simulink model "six_plus_six_AcmsteeringV09_main"  (R2014a)
settings: Solver=FixedStepDiscrete  StartTime=0.0  StopTime=10.0  FixedStep=0.0005  RelTol=1e-3
InitFcn:
  | Veh_Par_wxt
values from neighbouring files (symbols this model uses):
  acc_spdctl = [0 100]    [Veh_Par_wxt.m]
  ag_thr = ecucoder_cal(ag_thr)    [Veh_Par_wxt.m]
  B = 1.8    [Veh_Par_wxt.m]
  bra_em = 100    [Veh_Par_wxt.m]
  bra_pre_gz2 = 100/3    (= 33.3333333333)    [Veh_Par_wxt.m]
  bra_pre_gz34 = 10/3    (= 3.33333333333)    [Veh_Par_wxt.m]
  bra_pre_yd = 10/2    (= 5)    [Veh_Par_wxt.m]
  brakepre_dem_data = [0 1 2 3 4 5 6 7 8 9 10]    [Veh_Par_wxt.m]
  brakeTrq_dem_data = [0 125 251 376 502 627 753 878 1004 1129 1255]    [Veh_Par_wxt.m]
  bratrq_max = 4*1255    (= 5020)    [Veh_Par_wxt.m]
  eff_tran = 0.9    [Veh_Par_wxt.m]
  ESP_switch = ecucoder_cal(ESP_switch)    [Veh_Par_wxt.m]
  G = Mass*g    (= 15696)    [Veh_Par_wxt.m]
  kd1 = ecucoder_cal(kd1)    [Veh_Par_wxt.m]
  kd2 = 0    [Veh_Par_wxt.m]
  ki1 = ecucoder_cal(ki1)    [Veh_Par_wxt.m]
  ki2 = 1    [Veh_Par_wxt.m]
  kp1 = ecucoder_cal(kp1)    [Veh_Par_wxt.m]
  kp2 = 300    [Veh_Par_wxt.m]
  L = L1+L2    (= 2.9)    [Veh_Par_wxt.m]
  premax = 100    [Veh_Par_wxt.m]
  Radius = 0.4572/2    (= 0.2286)    [Veh_Par_wxt.m]
  RC_switch = ecucoder_cal(RC_switch)    [Veh_Par_wxt.m]
  s_opt_yi = 0.15    [Veh_Par_wxt.m]
  s_opt_zhuan = 0.8    [Veh_Par_wxt.m]
  s_opt_zhuan_add = 0.05    [Veh_Par_wxt.m]
  s_opt_zhuan_table = [0.8 0.8 0.3 0.3]    [Veh_Par_wxt.m]
  spd_map_mot = [0 499.85 999.79 1500 2000 2500 3000 3500 4000 4500 4999.8 5999.8]    [Veh_Par_wxt.m]
  spd_spdctl = [0 500]    [Veh_Par_wxt.m]
  speed_thr_park = 5/3.6/Radius*tras_ratio*30/pi    (= 464.143899364)    [Veh_Par_wxt.m]
  TCS_switch = ecucoder_cal(TCS_switch)    [Veh_Par_wxt.m]
  tras_ratio = 8    [Veh_Par_wxt.m]
  trq_map_mot = [70.5 70.012 71.154 65.797 53.917 45.159 38.073 32.685 27.48 17.133 14.949 10.07]    [Veh_Par_wxt.m]
  trqmax_yd = 70.5    [Veh_Par_wxt.m]
  trqmax_zx = 70.5    [Veh_Par_wxt.m]
  trqmaxneg = -70.5    [Veh_Par_wxt.m]
  v_gain = 0.9    [Veh_Par_wxt.m]
  v_table = [0 5 20 100]    [Veh_Par_wxt.m]
  v_thr_park = 5    [Veh_Par_wxt.m]
  zhidong_bianmazhi = [-140000 750000]    [Veh_Par_wxt.m]
  zhidong_down = -140000    [Veh_Par_wxt.m]
  zhidong_up = 750000    [Veh_Par_wxt.m]
  zhidong_youmen = [0 100]    [Veh_Par_wxt.m]
  zhuanxiang_bianmazhi = [-400000 0 400000]    [Veh_Par_wxt.m]
  zhuanxiang_down = -400000    [Veh_Par_wxt.m]
  zhuanxiang_up = 400000    [Veh_Par_wxt.m]
  zhuanxiang_youmen = [-100 0 100]    [Veh_Par_wxt.m]
undefined symbols (not defined in the file or in its folder): ecucoder_acal, guzhang_lf, guzhang_lm, guzhang_lr, guzhang_rf, guzhang_rm, guzhang_rr, myFIS
libraries: simulink x979, ec5744lib x59, fuzblock x2
(part 16 of 26)

== system six_plus_six_AcmsteeringV09_main/Subsystem/VCU4/VCU1_GearCmd ==
  VCU1_GearCmd : Inport
  Constant{2..8} (7 alike) : Constant  Value=0  OutDataTypeStr=uint8
  VCU1_GearCmdRon : Rounding  Operator=round
  VCU1_GearCmd_1sat : Saturate  UpperLimit=24  LowerLimit=0
  VCU1_GearCmd_Convert : DataTypeConversion  OutDataTypeStr=uint8
  VCU1_GearCmd_Convert1 : DataTypeConversion  OutDataTypeStr=uint32
  VCU1_GearCmd_D : Product  Inputs=*/
  VCU1_GearCmd_F : Constant  OutDataTypeStr=single
  VCU1_GearCmd_L : simulink/Logic and Bit Operations/Bitwise Operator  logicop=AND  UseBitMask=on  BitMask=24  BitMaskRealWorld=Stored Integer
  VCU1_GearCmd_O : Constant  Value=0  OutDataTypeStr=single
  VCU1_GearCmd_S : ArithShift  BitShiftNumber=-3
  VCU1_GearCmd_sat : Saturate  UpperLimit=3  LowerLimit=0
  VCU1_GearCmd_st : Sum  Inputs=+-
  output1 : Outport
  output2 : Outport  Port=2
  output3 : Outport  Port=3
  output4 : Outport  Port=4
  output5 : Outport  Port=5
  output6 : Outport  Port=6
  output7 : Outport  Port=7
  output8 : Outport  Port=8
  wires:
  VCU1_GearCmd/1 -> VCU1_GearCmd_sat/1
  VCU1_GearCmd_sat/1 -> VCU1_GearCmd_st/1
  VCU1_GearCmd_O/1 -> VCU1_GearCmd_st/2
  VCU1_GearCmd_st/1 -> VCU1_GearCmd_D/1
  VCU1_GearCmd_F/1 -> VCU1_GearCmd_D/2
  VCU1_GearCmd_D/1 -> VCU1_GearCmdRon/1
  VCU1_GearCmdRon/1 -> VCU1_GearCmd_S/1
  VCU1_GearCmd_S/1 -> VCU1_GearCmd_1sat/1
  VCU1_GearCmd_1sat/1 -> VCU1_GearCmd_Convert1/1
  VCU1_GearCmd_Convert1/1 -> VCU1_GearCmd_L/1
  VCU1_GearCmd_L/1 -> VCU1_GearCmd_Convert/1
  VCU1_GearCmd_Convert/1 -> output1/1
  Constant2/1 -> output2/1
  Constant3/1 -> output3/1
  Constant4/1 -> output4/1
  Constant5/1 -> output5/1
  Constant6/1 -> output6/1
  Constant7/1 -> output7/1
  Constant8/1 -> output8/1

== system six_plus_six_AcmsteeringV09_main/Subsystem/VCU4/VCU1_LifeCnt ==
  VCU1_LifeCnt : Inport
  Constant{1..7} (7 alike) : Constant  Value=0  OutDataTypeStr=uint8
  VCU1_LifeCntRon : Rounding  Operator=round
  VCU1_LifeCnt_1sat : Saturate  UpperLimit=255  LowerLimit=0
  VCU1_LifeCnt_Convert : DataTypeConversion  OutDataTypeStr=uint8
  VCU1_LifeCnt_Convert1 : DataTypeConversion  OutDataTypeStr=uint32
  VCU1_LifeCnt_D : Product  Inputs=*/
  VCU1_LifeCnt_F : Constant  OutDataTypeStr=single
  VCU1_LifeCnt_L : simulink/Logic and Bit Operations/Bitwise Operator  logicop=AND  UseBitMask=on  BitMask=255  BitMaskRealWorld=Stored Integer
  VCU1_LifeCnt_O : Constant  Value=0  OutDataTypeStr=single
  VCU1_LifeCnt_S : ArithShift
  VCU1_LifeCnt_sat : Saturate  UpperLimit=255  LowerLimit=0
  VCU1_LifeCnt_st : Sum  Inputs=+-
  output1 : Outport
  output2 : Outport  Port=2
  output3 : Outport  Port=3
  output4 : Outport  Port=4
  output5 : Outport  Port=5
  output6 : Outport  Port=6
  output7 : Outport  Port=7
  output8 : Outport  Port=8
  wires:
  VCU1_LifeCnt/1 -> VCU1_LifeCnt_sat/1
  VCU1_LifeCnt_sat/1 -> VCU1_LifeCnt_st/1
  VCU1_LifeCnt_O/1 -> VCU1_LifeCnt_st/2
  VCU1_LifeCnt_st/1 -> VCU1_LifeCnt_D/1
  VCU1_LifeCnt_F/1 -> VCU1_LifeCnt_D/2
  VCU1_LifeCnt_D/1 -> VCU1_LifeCntRon/1
  VCU1_LifeCntRon/1 -> VCU1_LifeCnt_S/1
  VCU1_LifeCnt_S/1 -> VCU1_LifeCnt_1sat/1
  VCU1_LifeCnt_1sat/1 -> VCU1_LifeCnt_Convert1/1
  VCU1_LifeCnt_Convert1/1 -> VCU1_LifeCnt_L/1
  VCU1_LifeCnt_L/1 -> VCU1_LifeCnt_Convert/1
  VCU1_LifeCnt_Convert/1 -> output8/1
  Constant1/1 -> output1/1
  Constant2/1 -> output2/1
  Constant3/1 -> output3/1
  Constant4/1 -> output4/1
  Constant5/1 -> output5/1
  Constant6/1 -> output6/1
  Constant7/1 -> output7/1

== system six_plus_six_AcmsteeringV09_main/Subsystem/VCU4/VCU1_SpeedMax ==
  VCU1_SpeedMax : Inport
  Constant{1,4..8} (6 alike) : Constant  Value=0  OutDataTypeStr=uint8
  VCU1_SpeedMaxBitCov : DataTypeConversion  OutDataTypeStr=uint8
  VCU1_SpeedMaxCOV : DataTypeConversion  OutDataTypeStr=uint8
  VCU1_SpeedMaxRon : Rounding  Operator=round
  VCU1_SpeedMax_1sat : Saturate  UpperLimit=65535  LowerLimit=0
  VCU1_SpeedMax_And : simulink/Logic and Bit Operations/Bitwise Operator  logicop=AND  UseBitMask=off  NumInputPorts=2  BitMask=bin2dec('11011001')  BitMaskRealWorld=Stored Integer
  VCU1_SpeedMax_And_C : Constant  Value=255  OutDataTypeStr=uint32
  VCU1_SpeedMax_Convert : DataTypeConversion  OutDataTypeStr=uint32
  VCU1_SpeedMax_D : Product  Inputs=*/
  VCU1_SpeedMax_D1 : Product  Inputs=*/
  VCU1_SpeedMax_F : Constant  OutDataTypeStr=single
  VCU1_SpeedMax_L : simulink/Logic and Bit Operations/Bitwise Operator  logicop=AND  UseBitMask=on  BitMask=65535  BitMaskRealWorld=Stored Integer
  VCU1_SpeedMax_O : Constant  Value=0  OutDataTypeStr=single
  VCU1_SpeedMax_S : ArithShift
  VCU1_SpeedMax_sat : Saturate  UpperLimit=10000  LowerLimit=0
  VCU1_SpeedMax_st : Sum  Inputs=+-
  VCU1_SpeedMaxoutput2_C : Constant  Value=256
  output1 : Outport
  output2 : Outport  Port=2
  output3 : Outport  Port=3
  output4 : Outport  Port=4
  output5 : Outport  Port=5
  output6 : Outport  Port=6
  output7 : Outport  Port=7
  output8 : Outport  Port=8
  wires:
  VCU1_SpeedMax/1 -> VCU1_SpeedMax_sat/1
  VCU1_SpeedMax_sat/1 -> VCU1_SpeedMax_st/1
  VCU1_SpeedMax_O/1 -> VCU1_SpeedMax_st/2
  VCU1_SpeedMax_st/1 -> VCU1_SpeedMax_D/1
  VCU1_SpeedMax_F/1 -> VCU1_SpeedMax_D/2
  VCU1_SpeedMax_D/1 -> VCU1_SpeedMaxRon/1
  VCU1_SpeedMaxRon/1 -> VCU1_SpeedMax_S/1
  VCU1_SpeedMax_S/1 -> VCU1_SpeedMax_1sat/1
  VCU1_SpeedMax_1sat/1 -> VCU1_SpeedMax_Convert/1
  VCU1_SpeedMax_Convert/1 -> VCU1_SpeedMax_L/1
  VCU1_SpeedMax_L/1 -> VCU1_SpeedMax_D1/1, VCU1_SpeedMax_And/1
  VCU1_SpeedMaxoutput2_C/1 -> VCU1_SpeedMax_D1/2
  VCU1_SpeedMax_D1/1 -> VCU1_SpeedMaxCOV/1
  VCU1_SpeedMaxCOV/1 -> output2/1
  VCU1_SpeedMax_And_C/1 -> VCU1_SpeedMax_And/2
  VCU1_SpeedMax_And/1 -> VCU1_SpeedMaxBitCov/1
  VCU1_SpeedMaxBitCov/1 -> output3/1
  Constant1/1 -> output1/1
  Constant4/1 -> output4/1
  Constant5/1 -> output5/1
  Constant6/1 -> output6/1
  Constant7/1 -> output7/1
  Constant8/1 -> output8/1

== system six_plus_six_AcmsteeringV09_main/Subsystem/VCU4/VCU1_TorqueRef ==
  VCU1_TorqueRef : Inport
  Constant{1..3,6..8} (6 alike) : Constant  Value=0  OutDataTypeStr=uint8
  VCU1_TorqueRefBitCov : DataTypeConversion  OutDataTypeStr=uint8
  VCU1_TorqueRefCOV : DataTypeConversion  OutDataTypeStr=uint8
  VCU1_TorqueRefRon : Rounding  Operator=round
  VCU1_TorqueRef_1sat : Saturate  UpperLimit=65535  LowerLimit=0
  VCU1_TorqueRef_And : simulink/Logic and Bit Operations/Bitwise Operator  logicop=AND  UseBitMask=off  NumInputPorts=2  BitMask=bin2dec('11011001')  BitMaskRealWorld=Stored Integer
  VCU1_TorqueRef_And_C : Constant  Value=255  OutDataTypeStr=uint32
  VCU1_TorqueRef_Convert : DataTypeConversion  OutDataTypeStr=uint32
  VCU1_TorqueRef_D : Product  Inputs=*/
  VCU1_TorqueRef_D1 : Product  Inputs=*/
  VCU1_TorqueRef_F : Constant  Value=0.1  OutDataTypeStr=single
  VCU1_TorqueRef_L : simulink/Logic and Bit Operations/Bitwise Operator  logicop=AND  UseBitMask=on  BitMask=65535  BitMaskRealWorld=Stored Integer
  VCU1_TorqueRef_O : Constant  Value=-1000  OutDataTypeStr=single
  VCU1_TorqueRef_S : ArithShift
  VCU1_TorqueRef_sat : Saturate  UpperLimit=1000  LowerLimit=-1000
  VCU1_TorqueRef_st : Sum  Inputs=+-
  VCU1_TorqueRefoutput4_C : Constant  Value=256
  output1 : Outport
  output2 : Outport  Port=2
  output3 : Outport  Port=3
  output4 : Outport  Port=4
  output5 : Outport  Port=5
  output6 : Outport  Port=6
  output7 : Outport  Port=7
  output8 : Outport  Port=8
  wires:
  VCU1_TorqueRef/1 -> VCU1_TorqueRef_sat/1
  VCU1_TorqueRef_sat/1 -> VCU1_TorqueRef_st/1
  VCU1_TorqueRef_O/1 -> VCU1_TorqueRef_st/2
  VCU1_TorqueRef_st/1 -> VCU1_TorqueRef_D/1
  VCU1_TorqueRef_F/1 -> VCU1_TorqueRef_D/2
  VCU1_TorqueRef_D/1 -> VCU1_TorqueRefRon/1
  VCU1_TorqueRefRon/1 -> VCU1_TorqueRef_S/1
  VCU1_TorqueRef_S/1 -> VCU1_TorqueRef_1sat/1
  VCU1_TorqueRef_1sat/1 -> VCU1_TorqueRef_Convert/1
  VCU1_TorqueRef_Convert/1 -> VCU1_TorqueRef_L/1
  VCU1_TorqueRef_L/1 -> VCU1_TorqueRef_D1/1, VCU1_TorqueRef_And/1
  VCU1_TorqueRefoutput4_C/1 -> VCU1_TorqueRef_D1/2
  VCU1_TorqueRef_D1/1 -> VCU1_TorqueRefCOV/1
  VCU1_TorqueRefCOV/1 -> output4/1
  VCU1_TorqueRef_And_C/1 -> VCU1_TorqueRef_And/2
  VCU1_TorqueRef_And/1 -> VCU1_TorqueRefBitCov/1
  VCU1_TorqueRefBitCov/1 -> output5/1
  Constant1/1 -> output1/1
  Constant2/1 -> output2/1
  Constant3/1 -> output3/1
  Constant6/1 -> output6/1
  Constant7/1 -> output7/1
  Constant8/1 -> output8/1

== system six_plus_six_AcmsteeringV09_main/Subsystem/VCU5/VCU1_CtrlModel ==
  VCU1_CtrlModel : Inport
  Constant{2..8} (7 alike) : Constant  Value=0  OutDataTypeStr=uint8
  VCU1_CtrlModelRon : Rounding  Operator=round
  VCU1_CtrlModel_1sat : Saturate  UpperLimit=4  LowerLimit=0
  VCU1_CtrlModel_Convert : DataTypeConversion  OutDataTypeStr=uint8
  VCU1_CtrlModel_Convert1 : DataTypeConversion  OutDataTypeStr=uint32
  VCU1_CtrlModel_D : Product  Inputs=*/
  VCU1_CtrlModel_F : Constant  OutDataTypeStr=single
  VCU1_CtrlModel_L : simulink/Logic and Bit Operations/Bitwise Operator  logicop=AND  UseBitMask=on  BitMask=4  BitMaskRealWorld=Stored Integer
  VCU1_CtrlModel_O : Constant  Value=0  OutDataTypeStr=single
  VCU1_CtrlModel_S : ArithShift  BitShiftNumber=-2
  VCU1_CtrlModel_sat : Saturate  UpperLimit=1  LowerLimit=0
  VCU1_CtrlModel_st : Sum  Inputs=+-
  output1 : Outport
  output2 : Outport  Port=2
  output3 : Outport  Port=3
  output4 : Outport  Port=4
  output5 : Outport  Port=5
  output6 : Outport  Port=6
  output7 : Outport  Port=7
  output8 : Outport  Port=8
  wires:
  VCU1_CtrlModel/1 -> VCU1_CtrlModel_sat/1
  VCU1_CtrlModel_sat/1 -> VCU1_CtrlModel_st/1
  VCU1_CtrlModel_O/1 -> VCU1_CtrlModel_st/2
  VCU1_CtrlModel_st/1 -> VCU1_CtrlModel_D/1
  VCU1_CtrlModel_F/1 -> VCU1_CtrlModel_D/2
  VCU1_CtrlModel_D/1 -> VCU1_CtrlModelRon/1
  VCU1_CtrlModelRon/1 -> VCU1_CtrlModel_S/1
  VCU1_CtrlModel_S/1 -> VCU1_CtrlModel_1sat/1
  VCU1_CtrlModel_1sat/1 -> VCU1_CtrlModel_Convert1/1
  VCU1_CtrlModel_Convert1/1 -> VCU1_CtrlModel_L/1
  VCU1_CtrlModel_L/1 -> VCU1_CtrlModel_Convert/1
  VCU1_CtrlModel_Convert/1 -> output1/1
  Constant2/1 -> output2/1
  Constant3/1 -> output3/1
  Constant4/1 -> output4/1
  Constant5/1 -> output5/1
  Constant6/1 -> output6/1
  Constant7/1 -> output7/1
  Constant8/1 -> output8/1

== system six_plus_six_AcmsteeringV09_main/Subsystem/VCU5/VCU1_EnableReq ==
  VCU1_EnableReq : Inport
  Constant{2..8} (7 alike) : Constant  Value=0  OutDataTypeStr=uint8
  VCU1_EnableReqRon : Rounding  Operator=round
  VCU1_EnableReq_1sat : Saturate  UpperLimit=3  LowerLimit=0
  VCU1_EnableReq_Convert : DataTypeConversion  OutDataTypeStr=uint8
  VCU1_EnableReq_Convert1 : DataTypeConversion  OutDataTypeStr=uint32
  VCU1_EnableReq_D : Product  Inputs=*/
  VCU1_EnableReq_F : Constant  OutDataTypeStr=single
  VCU1_EnableReq_L : simulink/Logic and Bit Operations/Bitwise Operator  logicop=AND  UseBitMask=on  BitMask=3  BitMaskRealWorld=Stored Integer
  VCU1_EnableReq_O : Constant  Value=0  OutDataTypeStr=single
  VCU1_EnableReq_S : ArithShift
  VCU1_EnableReq_sat : Saturate  UpperLimit=3  LowerLimit=0
  VCU1_EnableReq_st : Sum  Inputs=+-
  output1 : Outport
  output2 : Outport  Port=2
  output3 : Outport  Port=3
  output4 : Outport  Port=4
  output5 : Outport  Port=5
  output6 : Outport  Port=6
  output7 : Outport  Port=7
  output8 : Outport  Port=8
  wires:
  VCU1_EnableReq/1 -> VCU1_EnableReq_sat/1
  VCU1_EnableReq_sat/1 -> VCU1_EnableReq_st/1
  VCU1_EnableReq_O/1 -> VCU1_EnableReq_st/2
  VCU1_EnableReq_st/1 -> VCU1_EnableReq_D/1
  VCU1_EnableReq_F/1 -> VCU1_EnableReq_D/2
  VCU1_EnableReq_D/1 -> VCU1_EnableReqRon/1
  VCU1_EnableReqRon/1 -> VCU1_EnableReq_S/1
  VCU1_EnableReq_S/1 -> VCU1_EnableReq_1sat/1
  VCU1_EnableReq_1sat/1 -> VCU1_EnableReq_Convert1/1
  VCU1_EnableReq_Convert1/1 -> VCU1_EnableReq_L/1
  VCU1_EnableReq_L/1 -> VCU1_EnableReq_Convert/1
  VCU1_EnableReq_Convert/1 -> output1/1
  Constant2/1 -> output2/1
  Constant3/1 -> output3/1
  Constant4/1 -> output4/1
  Constant5/1 -> output5/1
  Constant6/1 -> output6/1
  Constant7/1 -> output7/1
  Constant8/1 -> output8/1

== system six_plus_six_AcmsteeringV09_main/Subsystem/VCU5/VCU1_GearCmd ==
  VCU1_GearCmd : Inport
  Constant{2..8} (7 alike) : Constant  Value=0  OutDataTypeStr=uint8
  VCU1_GearCmdRon : Rounding  Operator=round
  VCU1_GearCmd_1sat : Saturate  UpperLimit=24  LowerLimit=0
  VCU1_GearCmd_Convert : DataTypeConversion  OutDataTypeStr=uint8
  VCU1_GearCmd_Convert1 : DataTypeConversion  OutDataTypeStr=uint32
  VCU1_GearCmd_D : Product  Inputs=*/
  VCU1_GearCmd_F : Constant  OutDataTypeStr=single
  VCU1_GearCmd_L : simulink/Logic and Bit Operations/Bitwise Operator  logicop=AND  UseBitMask=on  BitMask=24  BitMaskRealWorld=Stored Integer
  VCU1_GearCmd_O : Constant  Value=0  OutDataTypeStr=single
  VCU1_GearCmd_S : ArithShift  BitShiftNumber=-3
  VCU1_GearCmd_sat : Saturate  UpperLimit=3  LowerLimit=0
  VCU1_GearCmd_st : Sum  Inputs=+-
  output1 : Outport
  output2 : Outport  Port=2
  output3 : Outport  Port=3
  output4 : Outport  Port=4
  output5 : Outport  Port=5
  output6 : Outport  Port=6
  output7 : Outport  Port=7
  output8 : Outport  Port=8
  wires:
  VCU1_GearCmd/1 -> VCU1_GearCmd_sat/1
  VCU1_GearCmd_sat/1 -> VCU1_GearCmd_st/1
  VCU1_GearCmd_O/1 -> VCU1_GearCmd_st/2
  VCU1_GearCmd_st/1 -> VCU1_GearCmd_D/1
  VCU1_GearCmd_F/1 -> VCU1_GearCmd_D/2
  VCU1_GearCmd_D/1 -> VCU1_GearCmdRon/1
  VCU1_GearCmdRon/1 -> VCU1_GearCmd_S/1
  VCU1_GearCmd_S/1 -> VCU1_GearCmd_1sat/1
  VCU1_GearCmd_1sat/1 -> VCU1_GearCmd_Convert1/1
  VCU1_GearCmd_Convert1/1 -> VCU1_GearCmd_L/1
  VCU1_GearCmd_L/1 -> VCU1_GearCmd_Convert/1
  VCU1_GearCmd_Convert/1 -> output1/1
  Constant2/1 -> output2/1
  Constant3/1 -> output3/1
  Constant4/1 -> output4/1
  Constant5/1 -> output5/1
  Constant6/1 -> output6/1
  Constant7/1 -> output7/1
  Constant8/1 -> output8/1

== system six_plus_six_AcmsteeringV09_main/Subsystem/VCU5/VCU1_LifeCnt ==
  VCU1_LifeCnt : Inport
  Constant{1..7} (7 alike) : Constant  Value=0  OutDataTypeStr=uint8
  VCU1_LifeCntRon : Rounding  Operator=round
  VCU1_LifeCnt_1sat : Saturate  UpperLimit=255  LowerLimit=0
  VCU1_LifeCnt_Convert : DataTypeConversion  OutDataTypeStr=uint8
  VCU1_LifeCnt_Convert1 : DataTypeConversion  OutDataTypeStr=uint32
  VCU1_LifeCnt_D : Product  Inputs=*/
  VCU1_LifeCnt_F : Constant  OutDataTypeStr=single
  VCU1_LifeCnt_L : simulink/Logic and Bit Operations/Bitwise Operator  logicop=AND  UseBitMask=on  BitMask=255  BitMaskRealWorld=Stored Integer
  VCU1_LifeCnt_O : Constant  Value=0  OutDataTypeStr=single
  VCU1_LifeCnt_S : ArithShift
  VCU1_LifeCnt_sat : Saturate  UpperLimit=255  LowerLimit=0
  VCU1_LifeCnt_st : Sum  Inputs=+-
  output1 : Outport
  output2 : Outport  Port=2
  output3 : Outport  Port=3
  output4 : Outport  Port=4
  output5 : Outport  Port=5
  output6 : Outport  Port=6
  output7 : Outport  Port=7
  output8 : Outport  Port=8
  wires:
  VCU1_LifeCnt/1 -> VCU1_LifeCnt_sat/1
  VCU1_LifeCnt_sat/1 -> VCU1_LifeCnt_st/1
  VCU1_LifeCnt_O/1 -> VCU1_LifeCnt_st/2
  VCU1_LifeCnt_st/1 -> VCU1_LifeCnt_D/1
  VCU1_LifeCnt_F/1 -> VCU1_LifeCnt_D/2
  VCU1_LifeCnt_D/1 -> VCU1_LifeCntRon/1
  VCU1_LifeCntRon/1 -> VCU1_LifeCnt_S/1
  VCU1_LifeCnt_S/1 -> VCU1_LifeCnt_1sat/1
  VCU1_LifeCnt_1sat/1 -> VCU1_LifeCnt_Convert1/1
  VCU1_LifeCnt_Convert1/1 -> VCU1_LifeCnt_L/1
  VCU1_LifeCnt_L/1 -> VCU1_LifeCnt_Convert/1
  VCU1_LifeCnt_Convert/1 -> output8/1
  Constant1/1 -> output1/1
  Constant2/1 -> output2/1
  Constant3/1 -> output3/1
  Constant4/1 -> output4/1
  Constant5/1 -> output5/1
  Constant6/1 -> output6/1
  Constant7/1 -> output7/1

== system six_plus_six_AcmsteeringV09_main/Subsystem/VCU5/VCU1_SpeedMax ==
  VCU1_SpeedMax : Inport
  Constant{1,4..8} (6 alike) : Constant  Value=0  OutDataTypeStr=uint8
  VCU1_SpeedMaxBitCov : DataTypeConversion  OutDataTypeStr=uint8
  VCU1_SpeedMaxCOV : DataTypeConversion  OutDataTypeStr=uint8
  VCU1_SpeedMaxRon : Rounding  Operator=round
  VCU1_SpeedMax_1sat : Saturate  UpperLimit=65535  LowerLimit=0
  VCU1_SpeedMax_And : simulink/Logic and Bit Operations/Bitwise Operator  logicop=AND  UseBitMask=off  NumInputPorts=2  BitMask=bin2dec('11011001')  BitMaskRealWorld=Stored Integer
  VCU1_SpeedMax_And_C : Constant  Value=255  OutDataTypeStr=uint32
  VCU1_SpeedMax_Convert : DataTypeConversion  OutDataTypeStr=uint32
  VCU1_SpeedMax_D : Product  Inputs=*/
  VCU1_SpeedMax_D1 : Product  Inputs=*/
  VCU1_SpeedMax_F : Constant  OutDataTypeStr=single
  VCU1_SpeedMax_L : simulink/Logic and Bit Operations/Bitwise Operator  logicop=AND  UseBitMask=on  BitMask=65535  BitMaskRealWorld=Stored Integer
  VCU1_SpeedMax_O : Constant  Value=0  OutDataTypeStr=single
  VCU1_SpeedMax_S : ArithShift
  VCU1_SpeedMax_sat : Saturate  UpperLimit=10000  LowerLimit=0
  VCU1_SpeedMax_st : Sum  Inputs=+-
  VCU1_SpeedMaxoutput2_C : Constant  Value=256
  output1 : Outport
  output2 : Outport  Port=2
  output3 : Outport  Port=3
  output4 : Outport  Port=4
  output5 : Outport  Port=5
  output6 : Outport  Port=6
  output7 : Outport  Port=7
  output8 : Outport  Port=8
  wires:
  VCU1_SpeedMax/1 -> VCU1_SpeedMax_sat/1
  VCU1_SpeedMax_sat/1 -> VCU1_SpeedMax_st/1
  VCU1_SpeedMax_O/1 -> VCU1_SpeedMax_st/2
  VCU1_SpeedMax_st/1 -> VCU1_SpeedMax_D/1
  VCU1_SpeedMax_F/1 -> VCU1_SpeedMax_D/2
  VCU1_SpeedMax_D/1 -> VCU1_SpeedMaxRon/1
  VCU1_SpeedMaxRon/1 -> VCU1_SpeedMax_S/1
  VCU1_SpeedMax_S/1 -> VCU1_SpeedMax_1sat/1
  VCU1_SpeedMax_1sat/1 -> VCU1_SpeedMax_Convert/1
  VCU1_SpeedMax_Convert/1 -> VCU1_SpeedMax_L/1
  VCU1_SpeedMax_L/1 -> VCU1_SpeedMax_D1/1, VCU1_SpeedMax_And/1
  VCU1_SpeedMaxoutput2_C/1 -> VCU1_SpeedMax_D1/2
  VCU1_SpeedMax_D1/1 -> VCU1_SpeedMaxCOV/1
  VCU1_SpeedMaxCOV/1 -> output2/1
  VCU1_SpeedMax_And_C/1 -> VCU1_SpeedMax_And/2
  VCU1_SpeedMax_And/1 -> VCU1_SpeedMaxBitCov/1
  VCU1_SpeedMaxBitCov/1 -> output3/1
  Constant1/1 -> output1/1
  Constant4/1 -> output4/1
  Constant5/1 -> output5/1
  Constant6/1 -> output6/1
  Constant7/1 -> output7/1
  Constant8/1 -> output8/1

== system six_plus_six_AcmsteeringV09_main/Subsystem/VCU5/VCU1_TorqueRef ==
  VCU1_TorqueRef : Inport
  Constant{1..3,6..8} (6 alike) : Constant  Value=0  OutDataTypeStr=uint8
  VCU1_TorqueRefBitCov : DataTypeConversion  OutDataTypeStr=uint8
  VCU1_TorqueRefCOV : DataTypeConversion  OutDataTypeStr=uint8
  VCU1_TorqueRefRon : Rounding  Operator=round
  VCU1_TorqueRef_1sat : Saturate  UpperLimit=65535  LowerLimit=0
  VCU1_TorqueRef_And : simulink/Logic and Bit Operations/Bitwise Operator  logicop=AND  UseBitMask=off  NumInputPorts=2  BitMask=bin2dec('11011001')  BitMaskRealWorld=Stored Integer
  VCU1_TorqueRef_And_C : Constant  Value=255  OutDataTypeStr=uint32
  VCU1_TorqueRef_Convert : DataTypeConversion  OutDataTypeStr=uint32
  VCU1_TorqueRef_D : Product  Inputs=*/
  VCU1_TorqueRef_D1 : Product  Inputs=*/
  VCU1_TorqueRef_F : Constant  Value=0.1  OutDataTypeStr=single
  VCU1_TorqueRef_L : simulink/Logic and Bit Operations/Bitwise Operator  logicop=AND  UseBitMask=on  BitMask=65535  BitMaskRealWorld=Stored Integer
  VCU1_TorqueRef_O : Constant  Value=-1000  OutDataTypeStr=single
  VCU1_TorqueRef_S : ArithShift
  VCU1_TorqueRef_sat : Saturate  UpperLimit=1000  LowerLimit=-1000
  VCU1_TorqueRef_st : Sum  Inputs=+-
  VCU1_TorqueRefoutput4_C : Constant  Value=256
  output1 : Outport
  output2 : Outport  Port=2
  output3 : Outport  Port=3
  output4 : Outport  Port=4
  output5 : Outport  Port=5
  output6 : Outport  Port=6
  output7 : Outport  Port=7
  output8 : Outport  Port=8
  wires:
  VCU1_TorqueRef/1 -> VCU1_TorqueRef_sat/1
  VCU1_TorqueRef_sat/1 -> VCU1_TorqueRef_st/1
  VCU1_TorqueRef_O/1 -> VCU1_TorqueRef_st/2
  VCU1_TorqueRef_st/1 -> VCU1_TorqueRef_D/1
  VCU1_TorqueRef_F/1 -> VCU1_TorqueRef_D/2
  VCU1_TorqueRef_D/1 -> VCU1_TorqueRefRon/1
  VCU1_TorqueRefRon/1 -> VCU1_TorqueRef_S/1
  VCU1_TorqueRef_S/1 -> VCU1_TorqueRef_1sat/1
  VCU1_TorqueRef_1sat/1 -> VCU1_TorqueRef_Convert/1
  VCU1_TorqueRef_Convert/1 -> VCU1_TorqueRef_L/1
  VCU1_TorqueRef_L/1 -> VCU1_TorqueRef_D1/1, VCU1_TorqueRef_And/1
  VCU1_TorqueRefoutput4_C/1 -> VCU1_TorqueRef_D1/2
  VCU1_TorqueRef_D1/1 -> VCU1_TorqueRefCOV/1
  VCU1_TorqueRefCOV/1 -> output4/1
  VCU1_TorqueRef_And_C/1 -> VCU1_TorqueRef_And/2
  VCU1_TorqueRef_And/1 -> VCU1_TorqueRefBitCov/1
  VCU1_TorqueRefBitCov/1 -> output5/1
  Constant1/1 -> output1/1
  Constant2/1 -> output2/1
  Constant3/1 -> output3/1
  Constant6/1 -> output6/1
  Constant7/1 -> output7/1
  Constant8/1 -> output8/1

== system six_plus_six_AcmsteeringV09_main/Subsystem/VCU6/VCU1_CtrlModel ==
  VCU1_CtrlModel : Inport
  Constant{2..8} (7 alike) : Constant  Value=0  OutDataTypeStr=uint8
  VCU1_CtrlModelRon : Rounding  Operator=round
  VCU1_CtrlModel_1sat : Saturate  UpperLimit=4  LowerLimit=0
  VCU1_CtrlModel_Convert : DataTypeConversion  OutDataTypeStr=uint8
  VCU1_CtrlModel_Convert1 : DataTypeConversion  OutDataTypeStr=uint32
  VCU1_CtrlModel_D : Product  Inputs=*/
  VCU1_CtrlModel_F : Constant  OutDataTypeStr=single
  VCU1_CtrlModel_L : simulink/Logic and Bit Operations/Bitwise Operator  logicop=AND  UseBitMask=on  BitMask=4  BitMaskRealWorld=Stored Integer
  VCU1_CtrlModel_O : Constant  Value=0  OutDataTypeStr=single
  VCU1_CtrlModel_S : ArithShift  BitShiftNumber=-2
  VCU1_CtrlModel_sat : Saturate  UpperLimit=1  LowerLimit=0
  VCU1_CtrlModel_st : Sum  Inputs=+-
  output1 : Outport
  output2 : Outport  Port=2
  output3 : Outport  Port=3
  output4 : Outport  Port=4
  output5 : Outport  Port=5
  output6 : Outport  Port=6
  output7 : Outport  Port=7
  output8 : Outport  Port=8
  wires:
  VCU1_CtrlModel/1 -> VCU1_CtrlModel_sat/1
  VCU1_CtrlModel_sat/1 -> VCU1_CtrlModel_st/1
  VCU1_CtrlModel_O/1 -> VCU1_CtrlModel_st/2
  VCU1_CtrlModel_st/1 -> VCU1_CtrlModel_D/1
  VCU1_CtrlModel_F/1 -> VCU1_CtrlModel_D/2
  VCU1_CtrlModel_D/1 -> VCU1_CtrlModelRon/1
  VCU1_CtrlModelRon/1 -> VCU1_CtrlModel_S/1
  VCU1_CtrlModel_S/1 -> VCU1_CtrlModel_1sat/1
  VCU1_CtrlModel_1sat/1 -> VCU1_CtrlModel_Convert1/1
  VCU1_CtrlModel_Convert1/1 -> VCU1_CtrlModel_L/1
  VCU1_CtrlModel_L/1 -> VCU1_CtrlModel_Convert/1
  VCU1_CtrlModel_Convert/1 -> output1/1
  Constant2/1 -> output2/1
  Constant3/1 -> output3/1
  Constant4/1 -> output4/1
  Constant5/1 -> output5/1
  Constant6/1 -> output6/1
  Constant7/1 -> output7/1
  Constant8/1 -> output8/1

== system six_plus_six_AcmsteeringV09_main/Subsystem/VCU6/VCU1_EnableReq ==
  VCU1_EnableReq : Inport
  Constant{2..8} (7 alike) : Constant  Value=0  OutDataTypeStr=uint8
  VCU1_EnableReqRon : Rounding  Operator=round
  VCU1_EnableReq_1sat : Saturate  UpperLimit=3  LowerLimit=0
  VCU1_EnableReq_Convert : DataTypeConversion  OutDataTypeStr=uint8
  VCU1_EnableReq_Convert1 : DataTypeConversion  OutDataTypeStr=uint32
  VCU1_EnableReq_D : Product  Inputs=*/
  VCU1_EnableReq_F : Constant  OutDataTypeStr=single
  VCU1_EnableReq_L : simulink/Logic and Bit Operations/Bitwise Operator  logicop=AND  UseBitMask=on  BitMask=3  BitMaskRealWorld=Stored Integer
  VCU1_EnableReq_O : Constant  Value=0  OutDataTypeStr=single
  VCU1_EnableReq_S : ArithShift
  VCU1_EnableReq_sat : Saturate  UpperLimit=3  LowerLimit=0
  VCU1_EnableReq_st : Sum  Inputs=+-
  output1 : Outport
  output2 : Outport  Port=2
  output3 : Outport  Port=3
  output4 : Outport  Port=4
  output5 : Outport  Port=5
  output6 : Outport  Port=6
  output7 : Outport  Port=7
  output8 : Outport  Port=8
  wires:
  VCU1_EnableReq/1 -> VCU1_EnableReq_sat/1
  VCU1_EnableReq_sat/1 -> VCU1_EnableReq_st/1
  VCU1_EnableReq_O/1 -> VCU1_EnableReq_st/2
  VCU1_EnableReq_st/1 -> VCU1_EnableReq_D/1
  VCU1_EnableReq_F/1 -> VCU1_EnableReq_D/2
  VCU1_EnableReq_D/1 -> VCU1_EnableReqRon/1
  VCU1_EnableReqRon/1 -> VCU1_EnableReq_S/1
  VCU1_EnableReq_S/1 -> VCU1_EnableReq_1sat/1
  VCU1_EnableReq_1sat/1 -> VCU1_EnableReq_Convert1/1
  VCU1_EnableReq_Convert1/1 -> VCU1_EnableReq_L/1
  VCU1_EnableReq_L/1 -> VCU1_EnableReq_Convert/1
  VCU1_EnableReq_Convert/1 -> output1/1
  Constant2/1 -> output2/1
  Constant3/1 -> output3/1
  Constant4/1 -> output4/1
  Constant5/1 -> output5/1
  Constant6/1 -> output6/1
  Constant7/1 -> output7/1
  Constant8/1 -> output8/1

== system six_plus_six_AcmsteeringV09_main/Subsystem/VCU6/VCU1_GearCmd ==
  VCU1_GearCmd : Inport
  Constant{2..8} (7 alike) : Constant  Value=0  OutDataTypeStr=uint8
  VCU1_GearCmdRon : Rounding  Operator=round
  VCU1_GearCmd_1sat : Saturate  UpperLimit=24  LowerLimit=0
  VCU1_GearCmd_Convert : DataTypeConversion  OutDataTypeStr=uint8
  VCU1_GearCmd_Convert1 : DataTypeConversion  OutDataTypeStr=uint32
  VCU1_GearCmd_D : Product  Inputs=*/
  VCU1_GearCmd_F : Constant  OutDataTypeStr=single
  VCU1_GearCmd_L : simulink/Logic and Bit Operations/Bitwise Operator  logicop=AND  UseBitMask=on  BitMask=24  BitMaskRealWorld=Stored Integer
  VCU1_GearCmd_O : Constant  Value=0  OutDataTypeStr=single
  VCU1_GearCmd_S : ArithShift  BitShiftNumber=-3
  VCU1_GearCmd_sat : Saturate  UpperLimit=3  LowerLimit=0
  VCU1_GearCmd_st : Sum  Inputs=+-
  output1 : Outport
  output2 : Outport  Port=2
  output3 : Outport  Port=3
  output4 : Outport  Port=4
  output5 : Outport  Port=5
  output6 : Outport  Port=6
  output7 : Outport  Port=7
  output8 : Outport  Port=8
  wires:
  VCU1_GearCmd/1 -> VCU1_GearCmd_sat/1
  VCU1_GearCmd_sat/1 -> VCU1_GearCmd_st/1
  VCU1_GearCmd_O/1 -> VCU1_GearCmd_st/2
  VCU1_GearCmd_st/1 -> VCU1_GearCmd_D/1
  VCU1_GearCmd_F/1 -> VCU1_GearCmd_D/2
  VCU1_GearCmd_D/1 -> VCU1_GearCmdRon/1
  VCU1_GearCmdRon/1 -> VCU1_GearCmd_S/1
  VCU1_GearCmd_S/1 -> VCU1_GearCmd_1sat/1
  VCU1_GearCmd_1sat/1 -> VCU1_GearCmd_Convert1/1
  VCU1_GearCmd_Convert1/1 -> VCU1_GearCmd_L/1
  VCU1_GearCmd_L/1 -> VCU1_GearCmd_Convert/1
  VCU1_GearCmd_Convert/1 -> output1/1
  Constant2/1 -> output2/1
  Constant3/1 -> output3/1
  Constant4/1 -> output4/1
  Constant5/1 -> output5/1
  Constant6/1 -> output6/1
  Constant7/1 -> output7/1
  Constant8/1 -> output8/1

== system six_plus_six_AcmsteeringV09_main/Subsystem/VCU6/VCU1_LifeCnt ==
  VCU1_LifeCnt : Inport
  Constant{1..7} (7 alike) : Constant  Value=0  OutDataTypeStr=uint8
  VCU1_LifeCntRon : Rounding  Operator=round
  VCU1_LifeCnt_1sat : Saturate  UpperLimit=255  LowerLimit=0
  VCU1_LifeCnt_Convert : DataTypeConversion  OutDataTypeStr=uint8
  VCU1_LifeCnt_Convert1 : DataTypeConversion  OutDataTypeStr=uint32
  VCU1_LifeCnt_D : Product  Inputs=*/
  VCU1_LifeCnt_F : Constant  OutDataTypeStr=single
  VCU1_LifeCnt_L : simulink/Logic and Bit Operations/Bitwise Operator  logicop=AND  UseBitMask=on  BitMask=255  BitMaskRealWorld=Stored Integer
  VCU1_LifeCnt_O : Constant  Value=0  OutDataTypeStr=single
  VCU1_LifeCnt_S : ArithShift
  VCU1_LifeCnt_sat : Saturate  UpperLimit=255  LowerLimit=0
  VCU1_LifeCnt_st : Sum  Inputs=+-
  output1 : Outport
  output2 : Outport  Port=2
  output3 : Outport  Port=3
  output4 : Outport  Port=4
  output5 : Outport  Port=5
  output6 : Outport  Port=6
  output7 : Outport  Port=7
  output8 : Outport  Port=8
  wires:
  VCU1_LifeCnt/1 -> VCU1_LifeCnt_sat/1
  VCU1_LifeCnt_sat/1 -> VCU1_LifeCnt_st/1
  VCU1_LifeCnt_O/1 -> VCU1_LifeCnt_st/2
  VCU1_LifeCnt_st/1 -> VCU1_LifeCnt_D/1
  VCU1_LifeCnt_F/1 -> VCU1_LifeCnt_D/2
  VCU1_LifeCnt_D/1 -> VCU1_LifeCntRon/1
  VCU1_LifeCntRon/1 -> VCU1_LifeCnt_S/1
  VCU1_LifeCnt_S/1 -> VCU1_LifeCnt_1sat/1
  VCU1_LifeCnt_1sat/1 -> VCU1_LifeCnt_Convert1/1
  VCU1_LifeCnt_Convert1/1 -> VCU1_LifeCnt_L/1
  VCU1_LifeCnt_L/1 -> VCU1_LifeCnt_Convert/1
  VCU1_LifeCnt_Convert/1 -> output8/1
  Constant1/1 -> output1/1
  Constant2/1 -> output2/1
  Constant3/1 -> output3/1
  Constant4/1 -> output4/1
  Constant5/1 -> output5/1
  Constant6/1 -> output6/1
  Constant7/1 -> output7/1

== system six_plus_six_AcmsteeringV09_main/Subsystem/VCU6/VCU1_SpeedMax ==
  VCU1_SpeedMax : Inport
  Constant{1,4..8} (6 alike) : Constant  Value=0  OutDataTypeStr=uint8
  VCU1_SpeedMaxBitCov : DataTypeConversion  OutDataTypeStr=uint8
  VCU1_SpeedMaxCOV : DataTypeConversion  OutDataTypeStr=uint8
  VCU1_SpeedMaxRon : Rounding  Operator=round
  VCU1_SpeedMax_1sat : Saturate  UpperLimit=65535  LowerLimit=0
  VCU1_SpeedMax_And : simulink/Logic and Bit Operations/Bitwise Operator  logicop=AND  UseBitMask=off  NumInputPorts=2  BitMask=bin2dec('11011001')  BitMaskRealWorld=Stored Integer
  VCU1_SpeedMax_And_C : Constant  Value=255  OutDataTypeStr=uint32
  VCU1_SpeedMax_Convert : DataTypeConversion  OutDataTypeStr=uint32
  VCU1_SpeedMax_D : Product  Inputs=*/
  VCU1_SpeedMax_D1 : Product  Inputs=*/
  VCU1_SpeedMax_F : Constant  OutDataTypeStr=single
  VCU1_SpeedMax_L : simulink/Logic and Bit Operations/Bitwise Operator  logicop=AND  UseBitMask=on  BitMask=65535  BitMaskRealWorld=Stored Integer
  VCU1_SpeedMax_O : Constant  Value=0  OutDataTypeStr=single
  VCU1_SpeedMax_S : ArithShift
  VCU1_SpeedMax_sat : Saturate  UpperLimit=10000  LowerLimit=0
  VCU1_SpeedMax_st : Sum  Inputs=+-
  VCU1_SpeedMaxoutput2_C : Constant  Value=256
  output1 : Outport
  output2 : Outport  Port=2
  output3 : Outport  Port=3
  output4 : Outport  Port=4
  output5 : Outport  Port=5
  output6 : Outport  Port=6
  output7 : Outport  Port=7
  output8 : Outport  Port=8
  wires:
  VCU1_SpeedMax/1 -> VCU1_SpeedMax_sat/1
  VCU1_SpeedMax_sat/1 -> VCU1_SpeedMax_st/1
  VCU1_SpeedMax_O/1 -> VCU1_SpeedMax_st/2
  VCU1_SpeedMax_st/1 -> VCU1_SpeedMax_D/1
  VCU1_SpeedMax_F/1 -> VCU1_SpeedMax_D/2
  VCU1_SpeedMax_D/1 -> VCU1_SpeedMaxRon/1
  VCU1_SpeedMaxRon/1 -> VCU1_SpeedMax_S/1
  VCU1_SpeedMax_S/1 -> VCU1_SpeedMax_1sat/1
  VCU1_SpeedMax_1sat/1 -> VCU1_SpeedMax_Convert/1
  VCU1_SpeedMax_Convert/1 -> VCU1_SpeedMax_L/1
  VCU1_SpeedMax_L/1 -> VCU1_SpeedMax_D1/1, VCU1_SpeedMax_And/1
  VCU1_SpeedMaxoutput2_C/1 -> VCU1_SpeedMax_D1/2
  VCU1_SpeedMax_D1/1 -> VCU1_SpeedMaxCOV/1
  VCU1_SpeedMaxCOV/1 -> output2/1
  VCU1_SpeedMax_And_C/1 -> VCU1_SpeedMax_And/2
  VCU1_SpeedMax_And/1 -> VCU1_SpeedMaxBitCov/1
  VCU1_SpeedMaxBitCov/1 -> output3/1
  Constant1/1 -> output1/1
  Constant4/1 -> output4/1
  Constant5/1 -> output5/1
  Constant6/1 -> output6/1
  Constant7/1 -> output7/1
  Constant8/1 -> output8/1

== system six_plus_six_AcmsteeringV09_main/Subsystem/VCU6/VCU1_TorqueRef ==
  VCU1_TorqueRef : Inport
  Constant{1..3,6..8} (6 alike) : Constant  Value=0  OutDataTypeStr=uint8
  VCU1_TorqueRefBitCov : DataTypeConversion  OutDataTypeStr=uint8
  VCU1_TorqueRefCOV : DataTypeConversion  OutDataTypeStr=uint8
  VCU1_TorqueRefRon : Rounding  Operator=round
  VCU1_TorqueRef_1sat : Saturate  UpperLimit=65535  LowerLimit=0
  VCU1_TorqueRef_And : simulink/Logic and Bit Operations/Bitwise Operator  logicop=AND  UseBitMask=off  NumInputPorts=2  BitMask=bin2dec('11011001')  BitMaskRealWorld=Stored Integer
  VCU1_TorqueRef_And_C : Constant  Value=255  OutDataTypeStr=uint32
  VCU1_TorqueRef_Convert : DataTypeConversion  OutDataTypeStr=uint32
  VCU1_TorqueRef_D : Product  Inputs=*/
  VCU1_TorqueRef_D1 : Product  Inputs=*/
  VCU1_TorqueRef_F : Constant  Value=0.1  OutDataTypeStr=single
  VCU1_TorqueRef_L : simulink/Logic and Bit Operations/Bitwise Operator  logicop=AND  UseBitMask=on  BitMask=65535  BitMaskRealWorld=Stored Integer
  VCU1_TorqueRef_O : Constant  Value=-1000  OutDataTypeStr=single
  VCU1_TorqueRef_S : ArithShift
  VCU1_TorqueRef_sat : Saturate  UpperLimit=1000  LowerLimit=-1000
  VCU1_TorqueRef_st : Sum  Inputs=+-
  VCU1_TorqueRefoutput4_C : Constant  Value=256
  output1 : Outport
  output2 : Outport  Port=2
  output3 : Outport  Port=3
  output4 : Outport  Port=4
  output5 : Outport  Port=5
  output6 : Outport  Port=6
  output7 : Outport  Port=7
  output8 : Outport  Port=8
  wires:
  VCU1_TorqueRef/1 -> VCU1_TorqueRef_sat/1
  VCU1_TorqueRef_sat/1 -> VCU1_TorqueRef_st/1
  VCU1_TorqueRef_O/1 -> VCU1_TorqueRef_st/2
  VCU1_TorqueRef_st/1 -> VCU1_TorqueRef_D/1
  VCU1_TorqueRef_F/1 -> VCU1_TorqueRef_D/2
  VCU1_TorqueRef_D/1 -> VCU1_TorqueRefRon/1
  VCU1_TorqueRefRon/1 -> VCU1_TorqueRef_S/1
  VCU1_TorqueRef_S/1 -> VCU1_TorqueRef_1sat/1
  VCU1_TorqueRef_1sat/1 -> VCU1_TorqueRef_Convert/1
  VCU1_TorqueRef_Convert/1 -> VCU1_TorqueRef_L/1
  VCU1_TorqueRef_L/1 -> VCU1_TorqueRef_D1/1, VCU1_TorqueRef_And/1
  VCU1_TorqueRefoutput4_C/1 -> VCU1_TorqueRef_D1/2
  VCU1_TorqueRef_D1/1 -> VCU1_TorqueRefCOV/1
  VCU1_TorqueRefCOV/1 -> output4/1
  VCU1_TorqueRef_And_C/1 -> VCU1_TorqueRef_And/2
  VCU1_TorqueRef_And/1 -> VCU1_TorqueRefBitCov/1
  VCU1_TorqueRefBitCov/1 -> output5/1
  Constant1/1 -> output1/1
  Constant2/1 -> output2/1
  Constant3/1 -> output3/1
  Constant6/1 -> output6/1
  Constant7/1 -> output7/1
  Constant8/1 -> output8/1

== system six_plus_six_AcmsteeringV09_main/Data_input/BMS1/BMS1/BMS1_SOC_Sub ==
  In1 : Inport
  Out1 : Outport
  wires:
  In1/1 -> Out1/1

== system six_plus_six_AcmsteeringV09_main/Data_input/BMS1/BMS1/BMS1_Sys_Status1_Sub ==
  In1 : Inport
  Out1 : Outport
  wires:
  In1/1 -> Out1/1

== system six_plus_six_AcmsteeringV09_main/Data_input/BMS1/BMS1/BMS1_Sys_Status2_Sub ==
  In1 : Inport
  Out1 : Outport
  wires:
  In1/1 -> Out1/1

== system six_plus_six_AcmsteeringV09_main/Data_input/BMS1/BMS1/BMS1_TotalCurrent_Sub ==
  In1 : Inport
  Out1 : Outport
  wires:
  In1/1 -> Out1/1

== system six_plus_six_AcmsteeringV09_main/Data_input/BMS1/BMS1/BMS1_TotalVol_Sub ==
  In1 : Inport
  Out1 : Outport
  wires:
  In1/1 -> Out1/1

== system six_plus_six_AcmsteeringV09_main/Data_input/BMS1-2/BMS1/BMS1_SOC_Sub ==
  In1 : Inport
  Out1 : Outport
  wires:
  In1/1 -> Out1/1

== system six_plus_six_AcmsteeringV09_main/Data_input/BMS1-2/BMS1/BMS1_Sys_Status1_Sub ==
  In1 : Inport
  Out1 : Outport
  wires:
  In1/1 -> Out1/1

== system six_plus_six_AcmsteeringV09_main/Data_input/BMS1-2/BMS1/BMS1_Sys_Status2_Sub ==
  In1 : Inport
  Out1 : Outport
  wires:
  In1/1 -> Out1/1

== system six_plus_six_AcmsteeringV09_main/Data_input/BMS1-2/BMS1/BMS1_TotalCurrent_Sub ==
  In1 : Inport
  Out1 : Outport
  wires:
  In1/1 -> Out1/1

== system six_plus_six_AcmsteeringV09_main/Data_input/BMS1-2/BMS1/BMS1_TotalVol_Sub ==
  In1 : Inport
  Out1 : Outport
  wires:
  In1/1 -> Out1/1

== system six_plus_six_AcmsteeringV09_main/Data_input/BMS1_1/BMS1/BMS1_SOC_Sub ==
  In1 : Inport
  Out1 : Outport
  wires:
  In1/1 -> Out1/1

== system six_plus_six_AcmsteeringV09_main/Data_input/BMS1_1/BMS1/BMS1_Sys_Status1_Sub ==
  In1 : Inport
  Out1 : Outport
  wires:
  In1/1 -> Out1/1

== system six_plus_six_AcmsteeringV09_main/Data_input/BMS1_1/BMS1/BMS1_Sys_Status2_Sub ==
  In1 : Inport
  Out1 : Outport
  wires:
  In1/1 -> Out1/1

== system six_plus_six_AcmsteeringV09_main/Data_input/BMS1_1/BMS1/BMS1_TotalCurrent_Sub ==
  In1 : Inport
  Out1 : Outport
  wires:
  In1/1 -> Out1/1

== system six_plus_six_AcmsteeringV09_main/Data_input/BMS1_1/BMS1/BMS1_TotalVol_Sub ==
  In1 : Inport
  Out1 : Outport
  wires:
  In1/1 -> Out1/1

== system six_plus_six_AcmsteeringV09_main/Data_input/BMS2/BMS2/BMS2_HighSingleVol_Sub ==
  In1 : Inport
  Out1 : Outport
  wires:
  In1/1 -> Out1/1

== system six_plus_six_AcmsteeringV09_main/Data_input/BMS2/BMS2/BMS2_LowSingleVol_Sub ==
  In1 : Inport
  Out1 : Outport
  wires:
  In1/1 -> Out1/1

== system six_plus_six_AcmsteeringV09_main/Data_input/BMS2_1/BMS2/BMS2_HighSingleVol_Sub ==
  In1 : Inport
  Out1 : Outport
  wires:
  In1/1 -> Out1/1

== system six_plus_six_AcmsteeringV09_main/Data_input/BMS2_1/BMS2/BMS2_LowSingleVol_Sub ==
  In1 : Inport
  Out1 : Outport
  wires:
  In1/1 -> Out1/1

== system six_plus_six_AcmsteeringV09_main/Data_input/BMS2_2/BMS2/BMS2_HighSingleVol_Sub ==
  In1 : Inport
  Out1 : Outport
  wires:
  In1/1 -> Out1/1

== system six_plus_six_AcmsteeringV09_main/Data_input/BMS2_2/BMS2/BMS2_LowSingleVol_Sub ==
  In1 : Inport
  Out1 : Outport
  wires:
  In1/1 -> Out1/1

== system six_plus_six_AcmsteeringV09_main/Data_input/BMS3/BMS3/BMS3_HighTemperature_Sub ==
  In1 : Inport
  Out1 : Outport
  wires:
  In1/1 -> Out1/1

== system six_plus_six_AcmsteeringV09_main/Data_input/BMS3/BMS3/BMS3_LowTemperature_Sub ==
  In1 : Inport
  Out1 : Outport
  wires:
  In1/1 -> Out1/1

== system six_plus_six_AcmsteeringV09_main/Data_input/BMS3_1/BMS3/BMS3_HighTemperature_Sub ==
  In1 : Inport
  Out1 : Outport
  wires:
  In1/1 -> Out1/1

== system six_plus_six_AcmsteeringV09_main/Data_input/BMS3_1/BMS3/BMS3_LowTemperature_Sub ==
  In1 : Inport
  Out1 : Outport
  wires:
  In1/1 -> Out1/1

== system six_plus_six_AcmsteeringV09_main/Data_input/BMS3_2/BMS3/BMS3_HighTemperature_Sub ==
  In1 : Inport
  Out1 : Outport
  wires:
  In1/1 -> Out1/1

== system six_plus_six_AcmsteeringV09_main/Data_input/BMS3_2/BMS3/BMS3_LowTemperature_Sub ==
  In1 : Inport
  Out1 : Outport
  wires:
  In1/1 -> Out1/1

== system six_plus_six_AcmsteeringV09_main/Data_input/BMS4/BMS4/BMS4_InputVolACC_Sub ==
  In1 : Inport
  Out1 : Outport
  wires:
  In1/1 -> Out1/1

== system six_plus_six_AcmsteeringV09_main/Data_input/BMS4/BMS4/BMS4_InputVolCHG_Sub ==
  In1 : Inport
  Out1 : Outport
  wires:
  In1/1 -> Out1/1

== system six_plus_six_AcmsteeringV09_main/Data_input/BMS4/BMS4/BMS4_InputVolKEYON_Sub ==
  In1 : Inport
  Out1 : Outport
  wires:
  In1/1 -> Out1/1

== system six_plus_six_AcmsteeringV09_main/Data_input/BMS4/BMS4/BMS4_Sys_Status3_Sub ==
  In1 : Inport
  Out1 : Outport
  wires:
  In1/1 -> Out1/1

== system six_plus_six_AcmsteeringV09_main/Data_input/BMS4_1/BMS4/BMS4_InputVolACC_Sub ==
  In1 : Inport
  Out1 : Outport
  wires:
  In1/1 -> Out1/1

== system six_plus_six_AcmsteeringV09_main/Data_input/BMS4_1/BMS4/BMS4_InputVolCHG_Sub ==
  In1 : Inport
  Out1 : Outport
  wires:
  In1/1 -> Out1/1

== system six_plus_six_AcmsteeringV09_main/Data_input/BMS4_1/BMS4/BMS4_InputVolKEYON_Sub ==
  In1 : Inport
  Out1 : Outport
  wires:
  In1/1 -> Out1/1

== system six_plus_six_AcmsteeringV09_main/Data_input/BMS4_1/BMS4/BMS4_Sys_Status3_Sub ==
  In1 : Inport
  Out1 : Outport
  wires:
  In1/1 -> Out1/1

== system six_plus_six_AcmsteeringV09_main/Data_input/BMS4_2/BMS4/BMS4_InputVolACC_Sub ==
  In1 : Inport
  Out1 : Outport
  wires:
  In1/1 -> Out1/1

== system six_plus_six_AcmsteeringV09_main/Data_input/BMS4_2/BMS4/BMS4_InputVolCHG_Sub ==
  In1 : Inport
  Out1 : Outport
  wires:
  In1/1 -> Out1/1

== system six_plus_six_AcmsteeringV09_main/Data_input/BMS4_2/BMS4/BMS4_InputVolKEYON_Sub ==
  In1 : Inport
  Out1 : Outport
  wires:
  In1/1 -> Out1/1

== system six_plus_six_AcmsteeringV09_main/Data_input/BMS4_2/BMS4/BMS4_Sys_Status3_Sub ==
  In1 : Inport
  Out1 : Outport
  wires:
  In1/1 -> Out1/1

== system six_plus_six_AcmsteeringV09_main/Data_input/BMS5/BMS5/BMS5_15s_InstanceDisPower_Sub ==
  In1 : Inport
  Out1 : Outport
  wires:
  In1/1 -> Out1/1

== system six_plus_six_AcmsteeringV09_main/Data_input/BMS5/BMS5/BMS5_ContDischargePower_Sub ==
  In1 : Inport
  Out1 : Outport
  wires:
  In1/1 -> Out1/1

== system six_plus_six_AcmsteeringV09_main/Data_input/BMS5/BMS5/BMS5_FailureLevel_Sub ==
  In1 : Inport
  Out1 : Outport
  wires:
  In1/1 -> Out1/1

== system six_plus_six_AcmsteeringV09_main/Data_input/BMS5/BMS5/BMS5_FeedbackPower_Sub ==
  In1 : Inport
  Out1 : Outport
  wires:
  In1/1 -> Out1/1

== system six_plus_six_AcmsteeringV09_main/Data_input/BMS5/BMS5/BMS5_UpDownRequest_Sub ==
  In1 : Inport
  Out1 : Outport
  wires:
  In1/1 -> Out1/1

== system six_plus_six_AcmsteeringV09_main/Data_input/BMS5_1/BMS5/BMS5_15s_InstanceDisPower_Sub ==
  In1 : Inport
  Out1 : Outport
  wires:
  In1/1 -> Out1/1

== system six_plus_six_AcmsteeringV09_main/Data_input/BMS5_1/BMS5/BMS5_ContDischargePower_Sub ==
  In1 : Inport
  Out1 : Outport
  wires:
  In1/1 -> Out1/1

== system six_plus_six_AcmsteeringV09_main/Data_input/BMS5_1/BMS5/BMS5_FailureLevel_Sub ==
  In1 : Inport
  Out1 : Outport
  wires:
  In1/1 -> Out1/1

== system six_plus_six_AcmsteeringV09_main/Data_input/BMS5_1/BMS5/BMS5_FeedbackPower_Sub ==
  In1 : Inport
  Out1 : Outport
  wires:
  In1/1 -> Out1/1

== system six_plus_six_AcmsteeringV09_main/Data_input/BMS5_1/BMS5/BMS5_UpDownRequest_Sub ==
  In1 : Inport
  Out1 : Outport
  wires:
  In1/1 -> Out1/1

== system six_plus_six_AcmsteeringV09_main/Data_input/BMS5_2/BMS5/BMS5_15s_InstanceDisPower_Sub ==
  In1 : Inport
  Out1 : Outport
  wires:
  In1/1 -> Out1/1

== system six_plus_six_AcmsteeringV09_main/Data_input/BMS5_2/BMS5/BMS5_ContDischargePower_Sub ==
  In1 : Inport
  Out1 : Outport
  wires:
  In1/1 -> Out1/1

== system six_plus_six_AcmsteeringV09_main/Data_input/BMS5_2/BMS5/BMS5_FailureLevel_Sub ==
  In1 : Inport
  Out1 : Outport
  wires:
  In1/1 -> Out1/1

== system six_plus_six_AcmsteeringV09_main/Data_input/BMS5_2/BMS5/BMS5_FeedbackPower_Sub ==
  In1 : Inport
  Out1 : Outport
  wires:
  In1/1 -> Out1/1

== system six_plus_six_AcmsteeringV09_main/Data_input/BMS5_2/BMS5/BMS5_UpDownRequest_Sub ==
  In1 : Inport
  Out1 : Outport
  wires:
  In1/1 -> Out1/1

== system six_plus_six_AcmsteeringV09_main/Data_input/MCU0/MCU0/MCU0_ControlMode_Sub ==
  In1 : Inport
  Out1 : Outport
  wires:
  In1/1 -> Out1/1

== system six_plus_six_AcmsteeringV09_main/Data_input/MCU0/MCU0/MCU0_EmergShutDown_Sub ==
  In1 : Inport
  Out1 : Outport
  wires:
  In1/1 -> Out1/1

== system six_plus_six_AcmsteeringV09_main/Data_input/MCU0/MCU0/MCU0_GearStatus_Sub ==
  In1 : Inport
  Out1 : Outport
  wires:
  In1/1 -> Out1/1

== system six_plus_six_AcmsteeringV09_main/Data_input/MCU0/MCU0/MCU0_HighVol_Sub ==
  In1 : Inport
  Out1 : Outport
  wires:
  In1/1 -> Out1/1

== matlab function six_plus_six_AcmsteeringV09_main/MainControl/mode_switch/mode_switch ==
  data: brake_emerg input; park input; mode_dem_out output int8; acc_dem input; steer_dem input; brake_dem input; center input; MCU0_SpeedFdk input; MCU0_1SpeedFdk input; MCU0_2SpeedFdk input; MCU0_3SpeedFdk input; MCU0_4SpeedFdk input; MCU0_5SpeedFdk input; speed_thr_park input; mode_dem_out_pre input
 function mode_dem_out = fcn(brake_emerg,park,acc_dem,steer_dem,brake_dem,center,MCU0_SpeedFdk,MCU0_1SpeedFdk,MCU0_2SpeedFdk,MCU0_3SpeedFdk,MCU0_4SpeedFdk,MCU0_5SpeedFdk,speed_thr_park,mode_dem_out_pre)
%#codegen
mode_dem_out=int8(mode_dem_out_pre);

if park==1  && MCU0_SpeedFdk<=speed_thr_park && MCU0_1SpeedFdk<=speed_thr_park && MCU0_2SpeedFdk<=speed_thr_park && MCU0_3SpeedFdk<=speed_thr_park  && MCU0_4SpeedFdk<=speed_thr_park  && MCU0_5SpeedFdk<=speed_thr_park && brake_emerg==0
    mode_dem_out=int8(0);
elseif acc_dem>0 && MCU0_SpeedFdk>=0 && MCU0_1SpeedFdk>=0 && MCU0_2SpeedFdk>=0 && MCU0_3SpeedFdk>=0  && MCU0_4SpeedFdk>=0  && MCU0_5SpeedFdk>=0 && brake_emerg==0  && park==0  && center==0
    mode_dem_out=int8(1);
elseif acc_dem==0 && brake_emerg==0  && park==0  && center==0
    mode_dem_out=int8(2);
elseif acc_dem<0 && MCU0_SpeedFdk>=0 && MCU0_1SpeedFdk>=0 && MCU0_2SpeedFdk>=0 && MCU0_3SpeedFdk>=0  && MCU0_4SpeedFdk>=0  && MCU0_5SpeedFdk>=0 && brake_emerg==0  && park==0  && center==0
    mode_dem_out=int8(3);
elseif center==1  && brake_emerg==0  && park==0        
    mode_dem_out=int8(4);
elseif brake_emerg==1
    mode_dem_out=int8(5);   
% else
%     mode_dem_out=int8(5);
end



end

== matlab function six_plus_six_AcmsteeringV09_main/MainControl/mode_control/Park/park/HeartBeat2 ==
  data: life_pre input; life output
function life = fcn(life_pre)
%#codegen
life=single(life_pre+1);
if life>255
    life=single(0);
end
end

== system six_plus_six_AcmsteeringV09_main/Data_input/MCU0/MCU0/MCU0_LiftCnt_Sub ==
  In1 : Inport
  Out1 : Outport
  wires:
  In1/1 -> Out1/1

== system six_plus_six_AcmsteeringV09_main/Data_input/MCU0/MCU0/MCU0_ShutDowAllow_Sub ==
  In1 : Inport
  Out1 : Outport
  wires:
  In1/1 -> Out1/1

== system six_plus_six_AcmsteeringV09_main/Data_input/MCU0/MCU0/MCU0_SpeedFdk_Sub ==
  In1 : Inport
  Out1 : Outport
  wires:
  In1/1 -> Out1/1

== system six_plus_six_AcmsteeringV09_main/Data_input/MCU0/MCU0/MCU0_TorqueFdk_Sub ==
  In1 : Inport
  Out1 : Outport
  wires:
  In1/1 -> Out1/1

== system six_plus_six_AcmsteeringV09_main/Data_input/MCU0/MCU0/MCU0_TorqueMax_Sub ==
  In1 : Inport
  Out1 : Outport
  wires:
  In1/1 -> Out1/1

== system six_plus_six_AcmsteeringV09_main/Data_input/MCU0/MCU0/MCU0_WorkStatus_Sub ==
  In1 : Inport
  Out1 : Outport
  wires:
  In1/1 -> Out1/1

== system six_plus_six_AcmsteeringV09_main/Data_input/MCU0_1/MCU0/MCU0_ControlMode_Sub ==
  In1 : Inport
  Out1 : Outport
  wires:
  In1/1 -> Out1/1

== system six_plus_six_AcmsteeringV09_main/Data_input/MCU0_1/MCU0/MCU0_EmergShutDown_Sub ==
  In1 : Inport
  Out1 : Outport
  wires:
  In1/1 -> Out1/1

== system six_plus_six_AcmsteeringV09_main/Data_input/MCU0_1/MCU0/MCU0_GearStatus_Sub ==
  In1 : Inport
  Out1 : Outport
  wires:
  In1/1 -> Out1/1

== system six_plus_six_AcmsteeringV09_main/Data_input/MCU0_1/MCU0/MCU0_HighVol_Sub ==
  In1 : Inport
  Out1 : Outport
  wires:
  In1/1 -> Out1/1

== system six_plus_six_AcmsteeringV09_main/Data_input/MCU0_1/MCU0/MCU0_LiftCnt_Sub ==
  In1 : Inport
  Out1 : Outport
  wires:
  In1/1 -> Out1/1

== system six_plus_six_AcmsteeringV09_main/Data_input/MCU0_1/MCU0/MCU0_ShutDowAllow_Sub ==
  In1 : Inport
  Out1 : Outport
  wires:
  In1/1 -> Out1/1

== system six_plus_six_AcmsteeringV09_main/Data_input/MCU0_1/MCU0/MCU0_SpeedFdk_Sub ==
  In1 : Inport
  Out1 : Outport
  wires:
  In1/1 -> Out1/1

== system six_plus_six_AcmsteeringV09_main/Data_input/MCU0_1/MCU0/MCU0_TorqueFdk_Sub ==
  In1 : Inport
  Out1 : Outport
  wires:
  In1/1 -> Out1/1

== system six_plus_six_AcmsteeringV09_main/Data_input/MCU0_1/MCU0/MCU0_TorqueMax_Sub ==
  In1 : Inport
  Out1 : Outport
  wires:
  In1/1 -> Out1/1

== system six_plus_six_AcmsteeringV09_main/Data_input/MCU0_1/MCU0/MCU0_WorkStatus_Sub ==
  In1 : Inport
  Out1 : Outport
  wires:
  In1/1 -> Out1/1

== system six_plus_six_AcmsteeringV09_main/Data_input/MCU0_2/MCU0/MCU0_ControlMode_Sub ==
  In1 : Inport
  Out1 : Outport
  wires:
  In1/1 -> Out1/1

== system six_plus_six_AcmsteeringV09_main/Data_input/MCU0_2/MCU0/MCU0_EmergShutDown_Sub ==
  In1 : Inport
  Out1 : Outport
  wires:
  In1/1 -> Out1/1

== system six_plus_six_AcmsteeringV09_main/Data_input/MCU0_2/MCU0/MCU0_GearStatus_Sub ==
  In1 : Inport
  Out1 : Outport
  wires:
  In1/1 -> Out1/1

== system six_plus_six_AcmsteeringV09_main/Data_input/MCU0_2/MCU0/MCU0_HighVol_Sub ==
  In1 : Inport
  Out1 : Outport
  wires:
  In1/1 -> Out1/1

== system six_plus_six_AcmsteeringV09_main/Data_input/MCU0_2/MCU0/MCU0_LiftCnt_Sub ==
  In1 : Inport
  Out1 : Outport
  wires:
  In1/1 -> Out1/1

== system six_plus_six_AcmsteeringV09_main/Data_input/MCU0_2/MCU0/MCU0_ShutDowAllow_Sub ==
  In1 : Inport
  Out1 : Outport
  wires:
  In1/1 -> Out1/1

== system six_plus_six_AcmsteeringV09_main/Data_input/MCU0_2/MCU0/MCU0_SpeedFdk_Sub ==
  In1 : Inport
  Out1 : Outport
  wires:
  In1/1 -> Out1/1

== system six_plus_six_AcmsteeringV09_main/Data_input/MCU0_2/MCU0/MCU0_TorqueFdk_Sub ==
  In1 : Inport
  Out1 : Outport
  wires:
  In1/1 -> Out1/1

== system six_plus_six_AcmsteeringV09_main/Data_input/MCU0_2/MCU0/MCU0_TorqueMax_Sub ==
  In1 : Inport
  Out1 : Outport
  wires:
  In1/1 -> Out1/1

== system six_plus_six_AcmsteeringV09_main/Data_input/MCU0_2/MCU0/MCU0_WorkStatus_Sub ==
  In1 : Inport
  Out1 : Outport
  wires:
  In1/1 -> Out1/1

== system six_plus_six_AcmsteeringV09_main/Data_input/MCU0_3/MCU0/MCU0_ControlMode_Sub ==
  In1 : Inport
  Out1 : Outport
  wires:
  In1/1 -> Out1/1

== system six_plus_six_AcmsteeringV09_main/Data_input/MCU0_3/MCU0/MCU0_EmergShutDown_Sub ==
  In1 : Inport
  Out1 : Outport
  wires:
  In1/1 -> Out1/1

== system six_plus_six_AcmsteeringV09_main/Data_input/MCU0_3/MCU0/MCU0_GearStatus_Sub ==
  In1 : Inport
  Out1 : Outport
  wires:
  In1/1 -> Out1/1
